simulink model "DroneControl_Bug2"  (R2020a)
settings: Solver=VariableStepAuto  StartTime=0.0  StopTime=65  RelTol=1e-3
values from neighbouring files (symbols this model uses):
  body_rate_0 = [0;0;0]    [Takeoff.m]
  Boundaries = [B1;B2;B3]    [Takeoff.m]
  Euler_0 = [0;0;0]    [Takeoff.m]
  g = [0;0;-9.8]    [Takeoff.m]
  m = m_drone + m_tank*percent    (= 36)    [Takeoff.m]    (also in animation.m = T_V1toI*T_V2toV1*T_BtoV2)
  MaxVel = 1.5    [Takeoff.m]
  MaxYawRate = 100*pi/180    (= 1.74532925199)    [Takeoff.m]
  RecObstacleYaw = [B1_Yaw,B2_Yaw,B3_Yaw]    [Takeoff.m]
  Target = WayPts(3,:)    [Takeoff.m]
  ts = 0.01    [Takeoff.m]
  WayPts = [[XYZ_0(1) XYZ_0(2) XYZ_0(3)] ... (first row only)    [Takeoff.m]
  XYZ_0 = [0;0;0]    [Takeoff.m]
undefined symbols (not defined in the file or in its folder): AccelGain, DiscIntNeverNeededParam, I
libraries: simulink x13, vrlib x2
(part 2 of 2)

== matlab function DroneControl_Bug2/Controller/Bug2_Rectangle Algorithm/CalCmd ==
  data: mode input; Target input; MaxVel input; SenseDist input; ObsYaw input; CalXbError output; XYZ input; CalYaw output
function [CalXbError,CalYaw] = fcn(mode,Target,MaxVel,SenseDist,ObsYaw,XYZ)
CalXbError = 0;
CalYaw = 0;
if mode == 0
    Xerror = Target(1) - XYZ(1);
    CalXbError = Xerror;
end

if abs(mode - 1) < 0.1
    Xerror = SenseDist - 1;
    CalXbError = Xerror;
end

if abs(mode - 2) < 0.1
    CalYaw = ObsYaw(1);
end

if abs(mode - 3) < 0.1
    CalXbError = MaxVel/0.6;
    CalYaw = ObsYaw(1);
end

if abs(mode -4) < 0.1
    CalYaw = ObsYaw(1);
end

if abs(mode - 5) < 0.1
    CalYaw = ObsYaw(2);
end

if abs(mode - 6) < 0.1
    CalXbError = MaxVel/0.6;
    CalYaw = ObsYaw(2);
end

if abs(mode - 7) < 0.1
    CalYaw = ObsYaw(2);
end

if abs(mode - 8) < 0.1
    CalYaw = ObsYaw(3);
end

if abs(mode - 9) < 0.1
    Xerror = Target(2) - XYZ(2);
    CalXbError = Xerror*1;
    CalYaw = ObsYaw(3);
end

if abs(mode - 10) < 0.1
    CalYaw = 0; % Dir from Target to Current XYZ.
end
 
if abs(mode - 11) < 0.1
    Xerror = Target(1) - XYZ(1);
    CalXbError = Xerror * 1;
    CalYaw = 0;
end



% 
% if abs(mode - 4) < 0.1
%     XTar = TarBound(1) + 1;
%     Xerror = XTar - XYZ(1);
%     CalXbError = Xerror * 1;
%     CalYaw = ObsYaw(2);
% end
% 
% if abs(mode - 5) < 0.1
%     CalYaw = ObsYaw(3);
% end
% 
% if abs(mode - 6) < 0.1
%     YTar = Target(2);
%     Yerror = Target(2) - XYZ(2);
%     CalXbError = 1*Yerror*1;
%     CalYaw = ObsYaw(3);
% end
% 
% if abs(mode - 7 ) < 0.1
%     CalXbError = 0;
%     CalYaw = 0;
% end
% 
% if abs(mode - 8) < 0.1
%     XTar = Target(1);
%     Xerror = XTar - XYZ(1);
%     CalXbError = Xerror * 1;
%     CalYaw = 0;
% end

== matlab function DroneControl_Bug2/6dof_system/BtoITransform ==
  data: phi input; m output; theta input; psi input
function m = fcn(phi,theta,psi)
    T_BtoV2 = [[1 0 0];[0 cos(-phi) sin(-phi)];[0 -sin(-phi) cos(-phi)]];
    T_V2toV1 = [[cos(-theta) 0 -sin(-theta)];[0 1 0];[sin(-theta) 0 cos(-theta)]];
    T_V1toI = [[cos(-psi) sin(-psi) 0];[-sin(-psi) cos(-psi) 0];[0 0 1]];
    m = T_V1toI*T_V2toV1*T_BtoV2;

== matlab function DroneControl_Bug2/6dof_system/euler_rate ==
  data: p input; phi_d output; q input; r input; phi input; theta input; theta_d output; psi_d output; psi input
function [phi_d,theta_d,psi_d] = fcn(p,q,r,phi,theta,psi)
    D = [[1 sin(phi)*tan(theta) cos(phi)*tan(theta)];
         [0 cos(phi) -sin(phi)];
         [0 sin(phi)/cos(theta) cos(phi)/cos(theta)]];
    euler_rate = D*[p;q;r]
    phi_d = euler_rate(1)
    theta_d = euler_rate(2)
    psi_d = euler_rate(3)

== matlab function DroneControl_Bug2/6dof_system/ItoBTransform ==
  data: phi input; m output; theta input; psi input
function m = fcn(phi,theta,psi)
    T_ItoV1 = [[cos(psi) sin(psi) 0];[-sin(psi) cos(psi) 0];[0 0 1]]; 
    T_V1toV2 = [[cos(theta) 0 -sin(theta)];[0 1 0];[sin(theta) 0 cos(theta)]];
    T_V2toB = [[1 0 0];[0 cos(phi) sin(phi)];[0 -sin(phi) cos(phi)]];
    m = T_V2toB*T_V1toV2*T_ItoV1

== matlab function DroneControl_Bug2/WayPts to XYZerror ==
  data: waypts input; XYZerror output; XYZ input
function XYZerror = fcn(waypts,XYZ)
Xerror = waypts(2,1)-XYZ(1);
Yerror = waypts(2,2)-XYZ(2);
Zerror = waypts(2,3)-XYZ(3);
XYZerror = [Xerror;Yerror;Zerror];

== matlab function DroneControl_Bug2/Controller/Bug2_Rectangle Algorithm/ChangeMode ==
  data: ObsYaw input; ForwardVel input; Yaw input; mode input; action output; SenseDist input; j input; Ye input
function action = fcn(ObsYaw,ForwardVel,Yaw,mode,SenseDist,j,Ye)
action = 0;

if mode == 0 && abs(SenseDist) < 3
    action = 1;
end

if abs(mode - 1) < 0.1 && abs(SenseDist-1) < 0.01
    action = 1;
end

if abs(mode - 2) < 0.1 && abs(Yaw-ObsYaw(1)) < 0.01
    action = 1;
end

if abs(mode - 3) < 0.1 && abs(SenseDist) > 0.7 && j < 0
    action = 1;
end

if abs(mode - 4) < 0.1 && abs(ForwardVel) < 0.1
    action = 1;
end

if abs(mode - 5) < 0.1 && abs(Yaw-ObsYaw(2)) < 0.01
    action = 1;
end

if abs(mode - 6) < 0.01 && abs(SenseDist) > 0.7 && j < 0
    action = 1;
end

if abs(mode - 7) < 0.01 && abs(ForwardVel) < 0.1
    action = 1;
end

if abs(mode - 8) < 0.01 && abs(Yaw-ObsYaw(3)) < 0.01
    action = 1;
end

if abs(mode - 9) < 0.01 && abs(Ye) < 0.01 && abs(ForwardVel) < 0.1
    action = 1;
end

if abs(mode - 10) < 0.01 && abs(Yaw-0) < 0.01
    action = 1;
end

== matlab function DroneControl_Bug2/Controller/Bug2_Rectangle Algorithm/MATLAB Function1 ==
  data: mode input; TarBound output; Boundaries input
function TarBound = fcn(mode,Boundaries)
if mode == 0
    TarBound = Boundaries(1,:);

elseif abs(mode - 1) < 0.1
    TarBound = Boundaries(1,:);
    
elseif abs(mode - 2) < 0.1
    TarBound = Boundaries(2,:);
    
elseif abs(mode - 3) < 0.1
    TarBound = Boundaries(2,:);
    
else
    TarBound = Boundaries(3,:);
    
end

== matlab function DroneControl_Bug2/Controller/Bug2_Rectangle Algorithm/MATLAB Function2 ==
  data: SensePt output; Pos input; Bound input; SenseDist output; j output
function [SensePt,SenseDist,j] = fcn(Pos,Bound)
if length(Bound) > 1
    bx = Bound(1);
    by = Bound(2);
    tx = Bound(3);
    ty = Bound(4);
    nx = Bound(5);
    ny = Bound(6);
    X = Pos(1);
    Y = Pos(2);
    Z = Pos(3);

    j = ((ty*bx-tx*by)-(ty*X-tx*Y))/(ty*nx-tx*ny);
    SensePt = [X+nx*j;Y+ny*j;Z+0];
    SenseDist = sqrt((nx*j)^2 + (ny*j)^2);
else
    SensePt = [0;0;0];
    SenseDist = 999;
    j = 999;
end
